simulink model "TestModelWLRover_Script"  (R2023a)
settings: Solver=ode4  StartTime=0.0  StopTime=10  FixedStep=0.0005  RelTol=1e-3
values from neighbouring files (symbols this model uses):
  ADAMS_cwd = 'C:\Users\wfism'    [Controls_Plant_2.m]
  ADAMS_exec = ''    [Controls_Plant_2.m]
  ADAMS_host = 'MSI'    [Controls_Plant_2.m]
  ADAMS_init = ''    [Controls_Plant_2.m]
  ADAMS_inputs = 'hipFLTorque!hipFRTorque!hipMLTorque!hipMRTorque!kneeFLTorque!kneeFRTorque!kneeMLTorque!kneeMRTorque!steerFLTorque!steerFRTorque!steerMLTorque!steerMRTorque!wheelFLTorque!wheelFRTorque!wheelMLTorque!wheelMRTorque'    [Controls_Plant_2.m]
  ADAMS_outputs = 'bodyAcceleration_X!bodyAcceleration_Y!bodyAcceleration_Z!bodyAngle_Pitch!bodyAngle_Roll!bodyAngle_Yaw!bodyAngVelocity_X!bodyAngVelocity_Y!bodyAngVelocity_Z!bodyCoord_X!bodyCoord_Y!bodyCoord_Z!bodyVelocity_X!bodyVelocity_Y!bodyVelocity_Z!hipFLAcceleration!hipFLAngle!hipFLSpeed!hipFRAcceleration!hipFRAngle!hipFRSpeed!hipMLAcceleration!hipMLAngle!hipMLSpeed!hipMRAcceleration!hipMRAngle!hipMRSpeed!kn ...(+718 chars)    [Controls_Plant_2.m]
  ADAMS_prefix = 'Controls_Plant_2'    [Controls_Plant_2.m]
  ADAMS_static = 'no'    [Controls_Plant_2.m]
  ADAMS_sysdir = 'C:\PROGRA~1\MSC~1.SOF\Adams\2019_2\'    [Controls_Plant_2.m]
undefined symbols (not defined in the file or in its folder): roverControllerScript, roverManager, stateWatcher
settings Model: SimulationMode=accelerator  Creator=i.shardyko  LastModifiedBy=a.abramenko
settings OptimizationCC: ReuseModelBlockBuffer=off

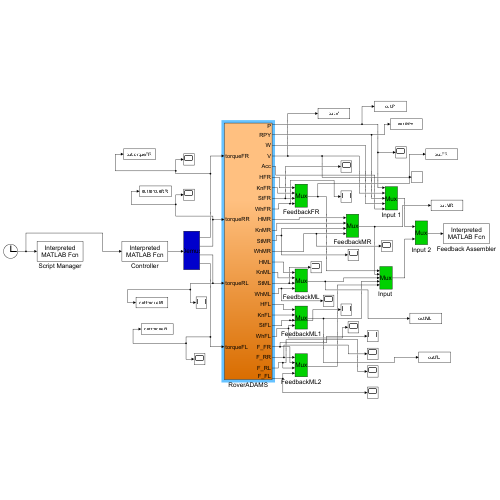
[thumbnail: Simulink's stored preview of the top-level diagram]
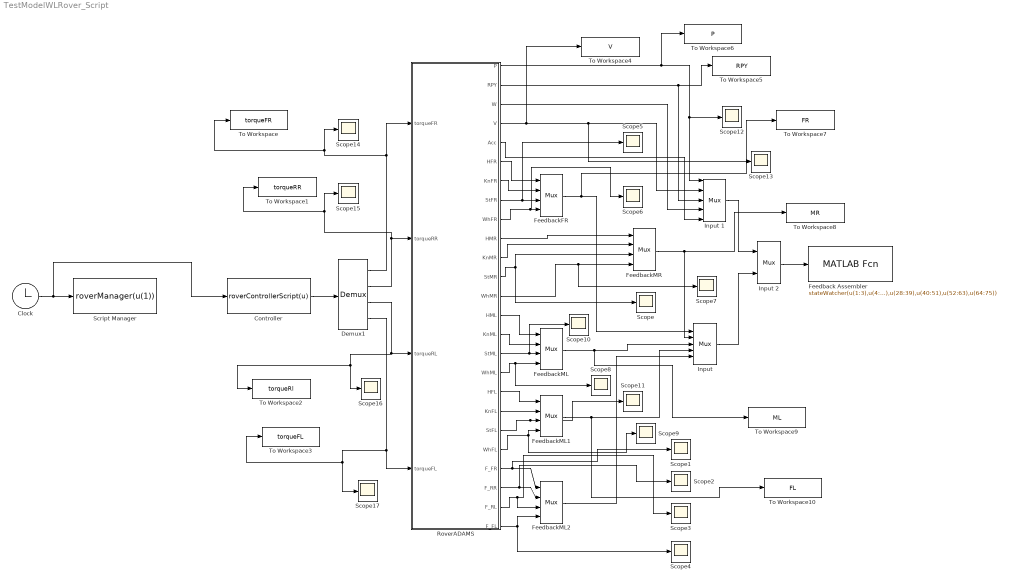
== system TestModelWLRover_Script ==
  Clock : Clock
  Controller : MATLABFcn  MATLABFcn=roverControllerScript(u)  OutputDimensions=16
  Demux1 : Demux
      settings: DisplayOption=none
  Feedback Assembler : MATLABFcn  MATLABFcn=stateWatcher(u(1:3),u(4:6),u(7:9),u(10:12),u(13:15),u(16:27),u(28:39),u(40:51),u(52:63),u(64:75))  OutputDimensions=0
  FeedbackFR : Mux
  FeedbackML : Mux
  FeedbackML1 : Mux
  FeedbackML2 : Mux
  FeedbackMR : Mux
  "Input " : Mux  Inputs=5
  Input 1 : Mux  Inputs=5
  Input 2 : Mux  Inputs=2
  RoverADAMS : Subsystem
  Scope{,1..17} (18 alike) : Scope
  Script Manager : MATLABFcn  MATLABFcn=roverManager(u(1))  OutputDimensions=0
  To Workspace : ToWorkspace  VariableName=torqueFR  SaveFormat=Timeseries  SampleTime=-1
  To Workspace1 : ToWorkspace  VariableName=torqueRR  SaveFormat=Timeseries  SampleTime=-1
  To Workspace10 : ToWorkspace  VariableName=FL  SaveFormat=Timeseries  SampleTime=-1
  To Workspace2 : ToWorkspace  VariableName=torqueRl  SaveFormat=Timeseries  SampleTime=-1
  To Workspace3 : ToWorkspace  VariableName=torqueFL  SaveFormat=Timeseries  SampleTime=-1
  To Workspace4 : ToWorkspace  VariableName=V  SaveFormat=Timeseries  SampleTime=-1
  To Workspace5 : ToWorkspace  VariableName=RPY  SaveFormat=Timeseries  SampleTime=-1
  To Workspace6 : ToWorkspace  VariableName=P  SaveFormat=Timeseries  SampleTime=-1
  To Workspace7 : ToWorkspace  VariableName=FR  SaveFormat=Timeseries  SampleTime=-1
  To Workspace8 : ToWorkspace  VariableName=MR  SaveFormat=Timeseries  SampleTime=-1
  To Workspace9 : ToWorkspace  VariableName=ML  SaveFormat=Timeseries  SampleTime=-1
  wires:
  Controller/1 -> Demux1/1
  Demux1/2 -> To Workspace1/1, Scope15/1, RoverADAMS/2(torqueRR)
  Demux1/3 -> To Workspace2/1, Scope16/1, RoverADAMS/3(torqueRL)
  Demux1/1 -> To Workspace/1, Scope14/1, RoverADAMS/1(torqueFR)
  Demux1/4 -> To Workspace3/1, Scope17/1, RoverADAMS/4(torqueFL)
  RoverADAMS/6(HFR) -> FeedbackFR/1
  RoverADAMS/7(KnFR) -> FeedbackFR/2
  RoverADAMS/8(StFR) -> Scope5/1, FeedbackFR/3
  RoverADAMS/9(WhFR) -> Scope6/1, FeedbackFR/4
  RoverADAMS/10(HMR) -> FeedbackMR/1
  RoverADAMS/11(KnMR) -> FeedbackMR/2
  RoverADAMS/12(StMR) -> FeedbackMR/3, Scope/1
  RoverADAMS/13(WhMR) -> Scope7/1, FeedbackMR/4
  FeedbackMR/1 -> To Workspace8/1, "Input "/2
  RoverADAMS/14(HML) -> FeedbackML/1
  RoverADAMS/15(KnML) -> FeedbackML/2
  RoverADAMS/16(StML) -> Scope10/1, FeedbackML/3
  RoverADAMS/17(WhML) -> FeedbackML/4, Scope8/1
  RoverADAMS/18(HFL) -> FeedbackML1/1
  RoverADAMS/19(KnFL) -> FeedbackML1/2
  RoverADAMS/20(StFL) -> Scope11/1, FeedbackML1/3
  RoverADAMS/21(WhFL) -> FeedbackML1/4, Scope9/1
  FeedbackML/1 -> To Workspace9/1, "Input "/3
  FeedbackML1/1 -> To Workspace10/1, "Input "/4
  RoverADAMS/22(F_FR) -> FeedbackML2/1, Scope1/1
  RoverADAMS/23(F_RR) -> Scope2/1, FeedbackML2/2
  RoverADAMS/24(F_RL) -> Scope3/1, FeedbackML2/3
  RoverADAMS/25(F_FL) -> FeedbackML2/4, Scope4/1
  FeedbackML2/1 -> "Input "/5
  FeedbackFR/1 -> To Workspace7/1, "Input "/1
  Clock/1 -> Controller/1, Script Manager/1
  Input 2/1 -> Feedback Assembler/1
  Input 1/1 -> Input 2/1
  "Input "/1 -> Input 2/2
  RoverADAMS/1(P) -> To Workspace6/1, Scope12/1, Input 1/1
  RoverADAMS/4(V) -> To Workspace4/1, Scope13/1, Input 1/2
  RoverADAMS/2(RPY) -> To Workspace5/1, Input 1/3
  RoverADAMS/3(W) -> Input 1/4
  RoverADAMS/5(Acc) -> Input 1/5

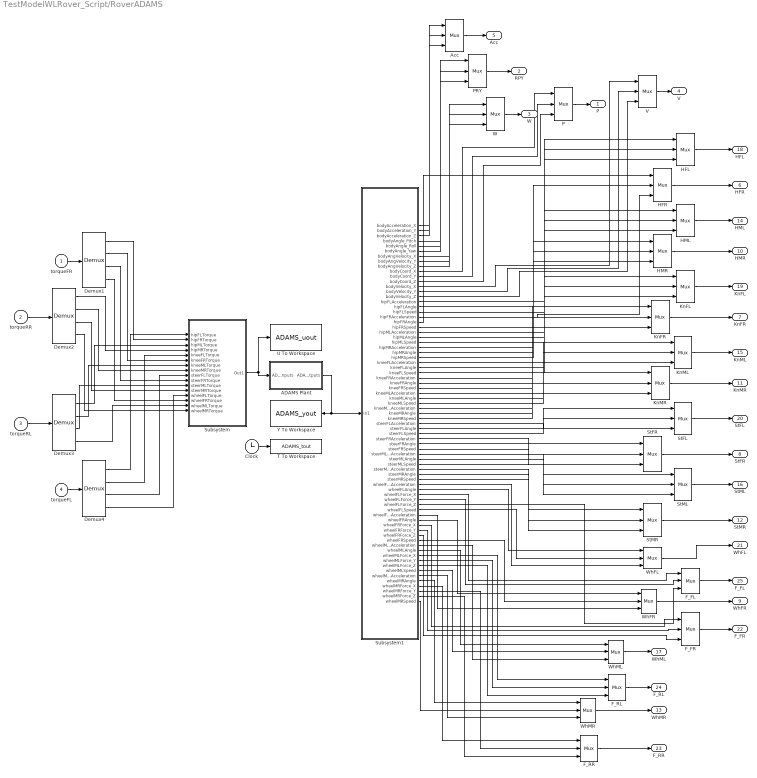
== system TestModelWLRover_Script/RoverADAMS ==
  torqueFR : Inport
  torqueRR : Inport  Port=2
  torqueRL : Inport  Port=3
  torqueFL : Inport  Port=4
  ADAMS Plant : Subsystem  LoadFcn=|  InitFcn=clear mex  mask(Adams Plant){exevie=ADAMS_sysdir, nam_in=ADAMS_inputs, namout=ADAMS_outputs, nampre=ADAMS_prefix, outfil=ADAMS_prefix, exesol=ADAMS_exec, stat=ADAMS_static, inicmd=[ADAMS_init], exetyp=C++, comtyp=PIPE(DDE), workdir=ADAMS_cwd, ada_host=ADAMS_host, modani=interactive, modsim=discrete, dft=no, simulink_lead_cosim=yes, pin_interp_order=0, pout_extrap_order=0, pin_extrap_order=0, pout_interp_order=0, dt_out=0.001, o_rate=1, more=off}
      | %check based on dialog box setting for when setting by popup menu                                             
      | if exist('ADAMS_solver_type')                                                                                 
      |   if strcmp(ADAMS_solver_type,'C++')                                                                          
      |     set_param(gcb,'exetyp','C++');                                                                            
      |   else                                                                                                        
      |     set_param(gcb,'exetyp','Fortran');                                                                        
      |   end                                                                                                         
      | else                                                                                                          
      |   set_param(gcb,'exetyp','C++');                                                                              
      | end                                                                                                           
      | %set the mode if using acar_solver                                                                            
      | %REQUIRED HERE BECAUSE BELOW CAUSES MDLTERMINATE TO BE CALLED 2 TIMES IN MIDDLE OF SIMULATION WHEN SET IN MASK
      |                                                                                                               
      | %enable the direct feedthrough, sim mode, anim mode parameters by default                                     
      |                                                                                                               
      | if exist('set_some_params_states')                                                                            
      |                                                                                                               
      |   set_some_params_states({'dft','modsim','modani'},{'on','on','on'},'MaskEnables',gcb)                        
      |   %turn on direct feedthrough option                                                                          
      |   set_some_params_states({'dft'},{'on'},'MaskVisibilities',gcb)                                               
      |                                                                                                               
      |  end                                                                                                          
      |                                                                                                               
      |                                                                                                               
      | if exist('ADAMS_exec')                                                                                        
      |   if and(strcmp(get_param(gcb,'exesol'),'ADAMS_exec'),strcmp(ADAMS_exec,'acar_solver'))                       
      |     %set the sim mode to discrete -- only supported mode                                                      
      |     set_param(gcb,'modsim','discrete')                                                                        
      |      %turn off direct feedthrough option                                                                      
      |      set_some_params_states({'dft'},{'off'},'MaskVisibilities',gcb)                                           
      |     %set the animation mode to batch -- only supported mode                                                   
      |     set_param(gcb,'modani','batch')                                                                           
      |     %disable the direct feedthrough, sim mode, anim mode parameters                                           
      |     set_some_params_states({'modsim','modani'},{'off','off'},'MaskEnables',gcb)                               
      |   end
      |   if and(strcmp(get_param(gcb,'exesol'),'ADAMS_exec'),strcmp(ADAMS_exec,'apre_solver'))                       
      |     %set the sim mode to discrete -- only supported mode                                                      
      |     set_param(gcb,'modsim','discrete')                                                                        
      |      %turn off direct feedthrough option                                                                      
      |      set_some_params_states({'dft'},{'off'},'MaskVisibilities',gcb)                                           
      |     %set the animation mode to batch -- only supported mode                                                   
      |     set_param(gcb,'modani','batch')                                                                           
      |     %disable the direct feedthrough, sim mode, anim mode parameters                                           
      |     set_some_params_states({'modsim','modani'},{'off','off'},'MaskEnables',gcb)                               
      |   end                                                                                                  
      | end
      mask prompts: exevie "Adams install directory"; nam_in "Adams View input names"; namout "Adams View output names"; nampre "Adams model file prefix"; outfil "Output files prefix (opt.: if blank - no output)"; exesol "User executable (opt.: if blank - use standard)"; stat "Initial static simulation flag"; inicmd "Initialization commands"; exetyp "Adams Solver type"; comtyp "Interprocess option"; workdir "Adams working directory"; ada_host "Adams host"; modani "Animation mode"; modsim "Simulation mode"; dft "Direct feedthrough"; simulink_lead_cosim "Discrete Computational Order - Simulink Leads Adams"; pin_interp_order "Plant input interpolation order"; pout_extrap_order "Plant output extrapolation order"; pin_extrap_order "Plant input extrapolation order"; pout_interp_order "Plant output interpolation order"; dt_out "Communication interval"; o_rate "Number of communications per output step"; more "More parameters"
      mask help: Simulate any Adams plant model either in Adams Solver form (.adm file) or in Adams View form (.cmd file)
      settings: OpenFcn=|
      | open_system(gcb,'mask')
      | if not(exist('set_some_params_states'))
      | 
      | warning('The script "set_some_params_states.m" cannot be found in the MATLAB PATH.  Cannot update the ADAMS Plant S-Function parameters.')
      | 
      | warning('Recommended action(optional):  run the Adams Controls .m file first to help choose the correct settings in the Adams S-Function block.')
      | 
      | end
      mask Help:
      | <html>
      | This S-Function represents the non-linear Adams Plant with the inputs sent to the Adams model <br>
      |  and the outputs generated by the Adams model.  See the Adams Controls documentation for more <br>
      | information.  This plant uses the following variables:<br>
      | <br>
      | <b>ADAMS_sysdir  :</b> Adams installation directory<br>
      | <b>ADAMS_inputs  :</b> Input variables View names vector<br>
      | <b>ADAMS_outputs :</b> Outputs variables View names vector<br>
      | <b>ADAMS_prefix  : </b>ADAMS model files prefix (.adm, .cmd); also doubles as output files prefix<br>
      | <b>ADAMS_exec :</b> Adams Solver user library or keyword (e.g., acar_solver)<br>
      | <b>ADAMS_static :</b> yes|no - initial static before Co-simulation(discrete)/Function Evaluation(continuous)<br>
      | <b>ADAMS_init :</b>Initialization commands (i.e., Adams View or Solver commands, depending on setting for Animation mode)<br>
      | <b>ADAMS_cwd : </b> Current working directory (for TCP/IP)<br>
      | <b>ADAMS_host : </b>Name of Adams server host (for TCP/IP)<br>
      | <b>ADAMS_mode :</b> Linear or non-linear (i.e., co-sim, function eval)<br>
      | <b>ADAMS_solver_type :</b>Fortran or C++ (used to set popup menu when first loaded) <br>
      | 
      | 
      | <br>
      | The following settings can be chosen:<br>
      | <br>
      | <b>Adams Solver type:</b>  Fortran or C++ (will also set ADAMS_solver_type)<br>
      | <b>Interprocess option:</b> Pipe(DDE), TCP/IP or DIRECT; TCP/IP can allow different machines run Adams and MATLAB<br>
      | <b>Animation mode:</b> batch (Solver, uses .adm) or interactive (View, uses .cmd)<br>
      | <b>Simulation mode:</b> discrete (Co-simulation) or continuous (Function Evaluation)<br>
      | <b>Discrete Computational Order - Simulink Lead Adams:</b> for discrete mode, chooses if Simulink leads the integration (yes) or lags (no);<br> if set to "no", can remove algebraic loop<br>
      | <b>Plant input interpolation order:</b> 0 = zero-order hold; 1 = linear (discrete mode only, where Simulink leads)<br>
      | <b>Plant output extrapolation order:</b> 0 = zero-order hold;1 = linear(discrete mode only, where Simulink leads)<br>
      | <b>Plant input extrapolation order:</b> 0 = zero-order hold; 1 = linear (discrete mode only, where Adams leads)<br>
      | <b>Plant output interpolation order:</b> 0 = zero-order hold;1 = linear(discrete mode only, where Adams leads)<br>
      | <b>Direct feedthrough:</b> yes|no - yes = Input directly effect output(continuous mode-only)<br>
      | <b>Communication interval:</b> Time step at which Co-simulation exchange information (e.g.,0.005); also controls <br>output for continuous mode (Function Evaluation)<br>
      | <b>Number of communications per output step: </b>Sets Adams output rate (.res, .req, .gra) integer value (default: 1)<br>
      | </html>
      mask Callback exesol:
      | if exist('set_some_params_states')
      | %enable the direct feedthrough, sim mode, anim mode parameters
      | set_some_params_states({'dft','modsim','modani'},{'on','on','on'},'MaskEnables',gcb)
      | %turn on direct feedthrough option
      | set_some_params_states({'dft'},{'on'},'MaskVisibilities',gcb)
      | end
      | 
      | if exist('ADAMS_exec')
      |   if and(strcmp(get_param(gcb,'exesol'),'ADAMS_exec'),strcmp(ADAMS_exec,'acar_solver'))
      |     %set the sim mode to discrete -- only supported mode
      |     %REMOVED:  BELOW CAUSES MDLTERMINATE TO BE CALLED 2 TIMES IN MIDDLE OF SIMULATION
      |     %Now in LoadFcn callback
      |     %set_param(gcb,'modsim','discrete')
      |      %turn off direct feedthrough option
      |     set_some_params_states({'dft'},{'off'},'MaskVisibilities',gcb)
      |     %set the animation mode to batch -- only supported mode
      |     %REMOVED:  BELOW CAUSES MDLTERMINATE TO BE CALLED 2 TIMES IN MIDDLE OF SIMULATION
      |     %Now in LoadFcn callback
      |     %set_param(gcb,'modani','batch')
      |     %disable the direct feedthrough, sim mode, anim mode parameters
      |     set_some_params_states({'modsim','modani'},{'off','off'},'MaskEnables',gcb)
      |   end
      | end
      mask TypeOptions exetyp: Fortran | C++
      mask Callback exetyp:
      | if strcmp(get_param(gcb,'exetyp'),'C++')
      |     ADAMS_solver_type='C++';
      | else
      |     ADAMS_solver_type='Fortran';
      | end
      mask TypeOptions comtyp: PIPE(DDE) | TCP/IP | DIRECT
      mask Callback comtyp:
      | if exist('set_some_params_states')
      | if strcmp(get_param(gcb,'comtyp'),'PIPE(DDE)') || strcmp(get_param(gcb,'comtyp'),'DIRECT')
      |     %turn off cwd, host options
      |     set_some_params_states({'ada_host','workdir'},{'off','off'},'MaskVisibilities',gcb)
      | else%if strcmp(get_param(gcb,'modsim'),'TCP/IP')
      |     %turn on cwd, host options
      |     set_some_params_states({'ada_host','workdir'},{'on','on'},'MaskVisibilities',gcb)
      | end
      | end
      mask TypeOptions modani: batch | interactive
      mask TypeOptions modsim: discrete | continuous
      mask Callback modsim:
      | if exist('set_some_params_states')
      | if strcmp(get_param(gcb,'modsim'),'discrete')
      |      %turn off direct feedthrough option
      |     set_some_params_states({'dft'},{'off'},'MaskVisibilities',gcb)
      |     %turn on discrete co-sim type if want to see more
      |     if strcmp(get_param(gcb,'more'),'on')
      |         set_some_params_states({'simulink_lead_cosim'},{'on'},'MaskVisibilities',gcb)
      |     end
      |     if strcmp(get_param(gcb,'simulink_lead_cosim'),'yes')
      |         %turn on interpolation/extrapolation options
      |         set_some_params_states({'pin_interp_order','pout_extrap_order',},{'on','on'},'MaskVisibilities',gcb)
      |     else
      |         set_some_params_states({'pin_extrap_order','pout_interp_order'},{'on','on'},'MaskVisibilities',gcb)
      |     end
      | else%if strcmp(get_param(gcb,'modsim'),'continuous')
      |      %turn off direct feedthrough option
      |     set_some_params_states({'dft'},{'on'},'MaskVisibilities',gcb)
      |     %turn off interpolation/extrapolation options
      |     set_some_params_states({'pin_interp_order','pout_extrap_order','pin_extrap_order','pout_interp_order','simulink_lead_cosim'},{'off','off','off','off','off'},'MaskVisibilities',gcb)
      | end
      | end
      mask TypeOptions dft: no | yes
      mask TypeOptions simulink_lead_cosim: yes | no
      mask Callback simulink_lead_cosim:
      | if exist('set_some_params_states')
      | if (strcmp(get_param(gcb,'simulink_lead_cosim'),'yes') && strcmp(get_param(gcb,'modsim'),'discrete'))
      |      %turn off unused interpolate/extrapolate options
      |     set_some_params_states({'pin_extrap_order','pout_interp_order'},{'off','off'},'MaskVisibilities',gcb)
      |     %turn on used interpolate/extrapolate options
      |     set_some_params_states({'pin_interp_order','pout_extrap_order'},{'on','on'},'MaskVisibilities',gcb)
      | elseif (strcmp(get_param(gcb,'simulink_lead_cosim'),'no') && strcmp(get_param(gcb,'modsim'),'discrete'))
      |     %turn on used interpolate/extrapolate options
      |     set_some_params_states({'pin_extrap_order','pout_interp_order'},{'on','on'},'MaskVisibilities',gcb)
      |      %turn off unused interpolate/extrapolate options
      |     set_some_params_states({'pin_interp_order','pout_extrap_order'},{'off','off'},'MaskVisibilities',gcb)
      | end
      | end
      mask TypeOptions pin_interp_order: 0 | 1
      mask TypeOptions pout_extrap_order: 0 | 1
      mask TypeOptions pin_extrap_order: 0 | 1
      mask TypeOptions pout_interp_order: 0 | 1
      mask Callback more:
      | if exist('set_some_params_states')
      | if (strcmp(get_param(gcb,'more'),'on'))
      |      %turn on infrequently used options
      |     set_some_params_states({'exevie','nam_in','namout','exesol','stat','inicmd'},{'on','on','on','on','on','on'},'MaskVisibilities',gcb)
      |     if strcmp(get_param(gcb,'modsim'),'discrete')
      |         set_some_params_states({'simulink_lead_cosim'},{'on'},'MaskVisibilities',gcb)
      |     end
      | elseif (strcmp(get_param(gcb,'more'),'off'))
      |     %turn off infrequently used options
      |     set_some_params_states({'exevie','nam_in','namout','exesol','stat','inicmd'},{'off','off','off','off','off','off'},'MaskVisibilities',gcb)
      |     if strcmp(get_param(gcb,'modsim'),'discrete')
      |         set_some_params_states({'simulink_lead_cosim'},{'off'},'MaskVisibilities',gcb)
      |     end
      | end
      | end
      mask Display: disp( 'MSC Software' )
  "Acc " : Mux  Inputs=3
  Clock : Clock
  Demux{1..4} (4 alike) : Demux
      settings: DisplayOption=none
  "F_FL " : Mux  Inputs=3
  "F_FR " : Mux  Inputs=3
  "F_RL " : Mux  Inputs=3
  "F_RR " : Mux  Inputs=3
  "HFL " : Mux  Inputs=3
  "HFR " : Mux  Inputs=3
  "HML " : Mux  Inputs=3
  "HMR " : Mux  Inputs=3
  "KnFL " : Mux  Inputs=3
  "KnFR " : Mux  Inputs=3
  "KnML " : Mux  Inputs=3
  "KnMR " : Mux  Inputs=3
  "P " : Mux  Inputs=3
  "PRY " : Mux  Inputs=3
  "StFL " : Mux  Inputs=3
  "StFR " : Mux  Inputs=3
  "StML " : Mux  Inputs=3
  "StMR " : Mux  Inputs=3
  Subsystem : Subsystem
  Subsystem1 : Subsystem
  T To Workspace : ToWorkspace  VariableName=ADAMS_tout
      settings: MaxDataPoints=100000
  U To Workspace : ToWorkspace  VariableName=ADAMS_uout
      settings: MaxDataPoints=100000
  "V " : Mux  Inputs=3
  "W " : Mux  Inputs=3
  "WhFL " : Mux  Inputs=3
  "WhFR " : Mux  Inputs=3
  "WhML " : Mux  Inputs=3
  "WhMR " : Mux  Inputs=3
  Y To Workspace : ToWorkspace  VariableName=ADAMS_yout
      settings: MaxDataPoints=100000
  P : Outport
  RPY : Outport  Port=2
  W : Outport  Port=3
  V : Outport  Port=4
  Acc : Outport  Port=5
  HFR : Outport  Port=6
  KnFR : Outport  Port=7
  StFR : Outport  Port=8
  WhFR : Outport  Port=9
  HMR : Outport  Port=10
  KnMR : Outport  Port=11
  StMR : Outport  Port=12
  WhMR : Outport  Port=13
  HML : Outport  Port=14
  KnML : Outport  Port=15
  StML : Outport  Port=16
  WhML : Outport  Port=17
  HFL : Outport  Port=18
  KnFL : Outport  Port=19
  StFL : Outport  Port=20
  WhFL : Outport  Port=21
  F_FR : Outport  Port=22
  F_RR : Outport  Port=23
  F_RL : Outport  Port=24
  F_FL : Outport  Port=25
  wires:
  Subsystem1/40(steerFLAcceleration) -> "StFL "/3
  Demux3/4 -> Subsystem/15(wheelMLTorque)
  Subsystem1/35("kneeMLAngle        ") -> "KnML "/1
  Subsystem1/38("kneeMRAngle        ") -> "KnMR "/1
  "HML "/1 -> HML/1
  Subsystem1/37("kneeMRAcceleration ") -> "KnMR "/3
  Demux2/1 -> Subsystem/4("hipMRTorque  ")
  Demux3/3 -> Subsystem/11(steerMLTorque)
  "StFR "/1 -> StFR/1
  Subsystem1/72("wheelMRForce_X     ") -> "F_RR "/1
  Subsystem1/74("wheelMRForce_Z     ") -> "F_RR "/3
  "StMR "/1 -> StMR/1
  "StFL "/1 -> StFL/1
  Subsystem1/70(wheelMRAcceleration) -> "WhMR "/3
  Subsystem1/65("wheelMLAngle       ") -> "WhML "/1
  Subsystem1/5("bodyAngle_Roll     ") -> "PRY "/2
  "HFL "/1 -> HFL/1
  Subsystem1/39("kneeMRSpeed        ") -> "KnMR "/2
  Subsystem1/51("steerMRSpeed       ") -> "StMR "/2
  Subsystem1/73("wheelMRForce_Y     ") -> "F_RR "/2
  Subsystem1/71("wheelMRAngle       ") -> "WhMR "/1
  torqueFR/1 -> Demux1/1
  "KnMR "/1 -> KnMR/1
  Clock/1 -> T To Workspace/1
  Subsystem1/42("steerFLSpeed       ") -> "StFL "/2
  torqueRL/1 -> Demux3/1
  Subsystem1/41("steerFLAngle       ") -> "StFL "/1
  Demux1/2 -> Subsystem/6("kneeFRTorque ")
  Subsystem1/63("wheelFRSpeed       ") -> "WhFR "/2
  Subsystem1/69("wheelMLSpeed       ") -> "WhML "/2
  Demux4/3 -> Subsystem/9(steerFLTorque)
  Demux1/1 -> Subsystem/2("hipFRTorque  ")
  Subsystem1/13("bodyVelocity_X     ") -> "V "/1
  Subsystem1/36("kneeMLSpeed        ") -> "KnML "/2
  Subsystem1/75("wheelMRSpeed       ") -> "WhMR "/2
  "WhML "/1 -> WhML/1
  Subsystem1/44("steerFRAngle       ") -> "StFR "/1
  Demux3/1 -> Subsystem/3("hipMLTorque  ")
  Subsystem1/56("wheelFLForce_Z     ") -> "F_FL "/3
  Demux4/1 -> Subsystem/1("hipFLTorque  ")
  Subsystem1/33("kneeFRSpeed        ") -> "KnFR "/2
  Subsystem1/27("hipMRSpeed         ") -> "HMR "/2
  Demux2/2 -> Subsystem/8("kneeMRTorque ")
  Demux3/2 -> Subsystem/7("kneeMLTorque ")
  "HFR "/1 -> HFR/1
  Subsystem/1(Out1) -> ADAMS Plant/1(ADAMS inputs), U To Workspace/1
  Subsystem1/59("wheelFRAngle       ") -> "WhFR "/1
  Demux1/3 -> Subsystem/10(steerFRTorque)
  Subsystem1/57("wheelFLSpeed       ") -> "WhFL "/2
  ADAMS Plant/1(ADAMS outputs) -> Subsystem1/1(In1), Y To Workspace/1
  Subsystem1/29("kneeFLAngle        ") -> "KnFL "/1
  Demux1/4 -> Subsystem/14(wheelFRTorque)
  Subsystem1/61("wheelFRForce_Y     ") -> "F_FR "/2
  "PRY "/1 -> RPY/1
  Demux2/4 -> Subsystem/16(wheelMRTorque)
  "KnML "/1 -> KnML/1
  Demux4/4 -> Subsystem/13(wheelFLTorque)
  Subsystem1/49(steerMRAcceleration) -> "StMR "/3
  "KnFR "/1 -> KnFR/1
  Subsystem1/62("wheelFRForce_Z     ") -> "F_FR "/3
  "WhFL "/1 -> WhFL/1
  Demux2/3 -> Subsystem/12(steerMRTorque)
  "P "/1 -> P/1
  Subsystem1/50("steerMRAngle       ") -> "StMR "/1
  "KnFL "/1 -> KnFL/1
  Subsystem1/32("kneeFRAngle        ") -> "KnFR "/1
  Subsystem1/28("kneeFLAcceleration ") -> "KnFL "/3
  Subsystem1/66("wheelMLForce_X     ") -> "F_RL "/1
  "V "/1 -> V/1
  Subsystem1/46(steerMLAcceleration) -> "StML "/3
  Subsystem1/58(wheelFRAcceleration) -> "WhFR "/3
  torqueRR/1 -> Demux2/1
  Subsystem1/67("wheelMLForce_Y     ") -> "F_RL "/2
  Subsystem1/64(wheelMLAcceleration) -> "WhML "/3
  Subsystem1/9("bodyAngVelocity_Z  ") -> "W "/3
  Subsystem1/14("bodyVelocity_Y     ") -> "V "/2
  Subsystem1/31("kneeFRAcceleration ") -> "KnFR "/3
  Subsystem1/8("bodyAngVelocity_Y  ") -> "W "/2
  Subsystem1/11("bodyCoord_Y        ") -> "P "/2
  Subsystem1/68("wheelMLForce_Z     ") -> "F_RL "/3
  Subsystem1/10("bodyCoord_X        ") -> "P "/1
  Subsystem1/12("bodyCoord_Z        ") -> "P "/3
  Subsystem1/4("bodyAngle_Pitch    ") -> "PRY "/1
  Subsystem1/24("hipMLSpeed         ") -> "HML "/2
  Subsystem1/26("hipMRAngle         ") -> "HMR "/1
  Subsystem1/55("wheelFLForce_Y     ") -> "F_FL "/2
  Subsystem1/60("wheelFRForce_X     ") -> "F_FR "/1
  Subsystem1/22("hipMLAcceleration  ") -> "HML "/3
  Subsystem1/34("kneeMLAcceleration ") -> "KnML "/3
  Subsystem1/23("hipMLAngle         ") -> "HML "/1
  Subsystem1/25("hipMRAcceleration  ") -> "HMR "/3
  Subsystem1/21("hipFRSpeed         ") -> "HFR "/2
  Subsystem1/20("hipFRAngle         ") -> "HFR "/1
  Subsystem1/53("wheelFLAngle       ") -> "WhFL "/1
  Subsystem1/47("steerMLAngle       ") -> "StML "/1
  Subsystem1/30("kneeFLSpeed        ") -> "KnFL "/2
  Subsystem1/17("hipFLAngle         ") -> "HFL "/1
  Subsystem1/19("hipFRAcceleration  ") -> "HFR "/3
  Subsystem1/18("hipFLSpeed         ") -> "HFL "/2
  Subsystem1/16("hipFLAcceleration  ") -> "HFL "/3
  Subsystem1/1("bodyAcceleration_X ") -> "Acc "/1
  Subsystem1/6("bodyAngle_Yaw      ") -> "PRY "/3
  Subsystem1/15("bodyVelocity_Z     ") -> "V "/3
  Subsystem1/7("bodyAngVelocity_X  ") -> "W "/1
  Subsystem1/3("bodyAcceleration_Z ") -> "Acc "/3
  Subsystem1/2("bodyAcceleration_Y ") -> "Acc "/2
  "Acc "/1 -> Acc/1
  Subsystem1/54("wheelFLForce_X     ") -> "F_FL "/1
  "WhFR "/1 -> WhFR/1
  Subsystem1/48("steerMLSpeed       ") -> "StML "/2
  torqueFL/1 -> Demux4/1
  "WhMR "/1 -> WhMR/1
  Subsystem1/52(wheelFLAcceleration) -> "WhFL "/3
  Subsystem1/43(steerFRAcceleration) -> "StFR "/3
  Subsystem1/45("steerFRSpeed       ") -> "StFR "/2
  Demux4/2 -> Subsystem/5("kneeFLTorque ")
  "StML "/1 -> StML/1
  "W "/1 -> W/1
  "HMR "/1 -> HMR/1
  "F_FR "/1 -> F_FR/1
  "F_RR "/1 -> F_RR/1
  "F_RL "/1 -> F_RL/1
  "F_FL "/1 -> F_FL/1

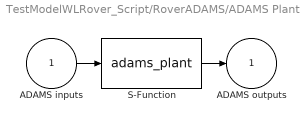
== system TestModelWLRover_Script/RoverADAMS/ADAMS Plant ==
  ADAMS inputs : Inport
  S-Function : S-Function  StopFcn=clear mex  FunctionName=adams_plant  Parameters=exevie,exesol,stat,outfil,nampre,o_rate,nam_in,namout,dft,modsim,modani,dt_out,inicmd,exetyp,comtyp,ada_host, workdir,pin_interp_order,pout_extrap_order,pin_extrap_order,pout_interp_order,simulink_lead_cosim  SFunctionDeploymentMode=off  EnableBusSupport=off
  ADAMS outputs : Outport  InitialOutput=0
  wires:
  ADAMS inputs/1 -> S-Function/1
  S-Function/1 -> ADAMS outputs/1

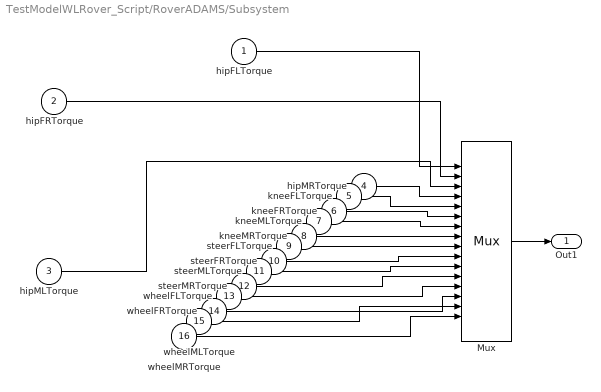
== system TestModelWLRover_Script/RoverADAMS/Subsystem ==
  "hipFLTorque  " : Inport
  "hipFRTorque  " : Inport  Port=2
  "hipMLTorque  " : Inport  Port=3
  "hipMRTorque  " : Inport  Port=4
  "kneeFLTorque " : Inport  Port=5
  "kneeFRTorque " : Inport  Port=6
  "kneeMLTorque " : Inport  Port=7
  "kneeMRTorque " : Inport  Port=8
  steerFLTorque : Inport  Port=9
  steerFRTorque : Inport  Port=10
  steerMLTorque : Inport  Port=11
  steerMRTorque : Inport  Port=12
  wheelFLTorque : Inport  Port=13
  wheelFRTorque : Inport  Port=14
  wheelMLTorque : Inport  Port=15
  wheelMRTorque : Inport  Port=16
  Mux : Mux  Inputs=16
  Out1 : Outport
  wires:
  "hipFLTorque  "/1 -> Mux/1
  "hipMRTorque  "/1 -> Mux/4
  "hipFRTorque  "/1 -> Mux/2
  steerMLTorque/1 -> Mux/11
  "kneeFLTorque "/1 -> Mux/5
  "kneeMRTorque "/1 -> Mux/8
  "kneeMLTorque "/1 -> Mux/7
  "kneeFRTorque "/1 -> Mux/6
  steerFLTorque/1 -> Mux/9
  wheelFLTorque/1 -> Mux/13
  steerFRTorque/1 -> Mux/10
  steerMRTorque/1 -> Mux/12
  wheelMLTorque/1 -> Mux/15
  "hipMLTorque  "/1 -> Mux/3
  wheelMRTorque/1 -> Mux/16
  wheelFRTorque/1 -> Mux/14
  Mux/1 -> Out1/1

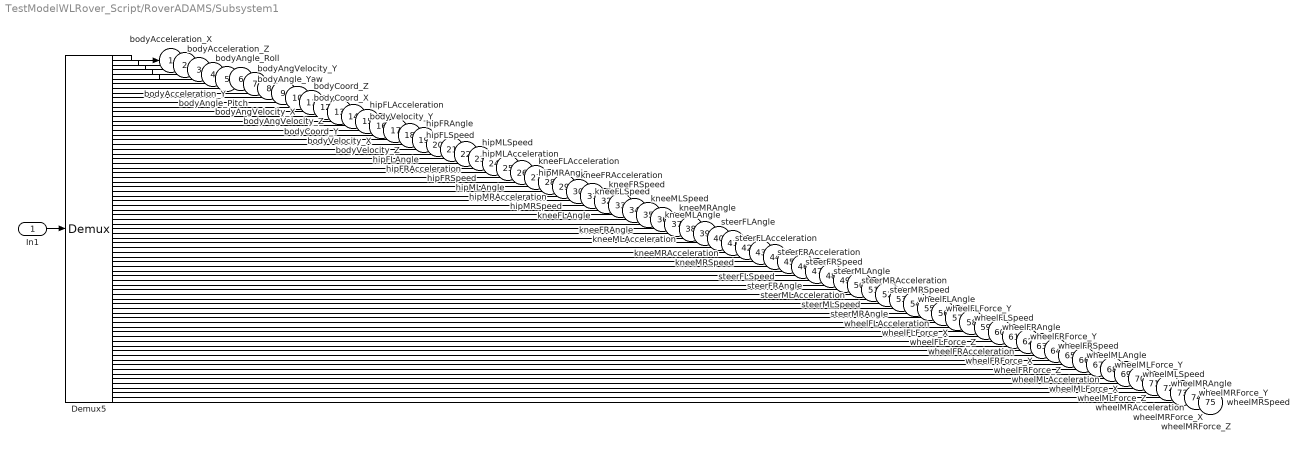
== system TestModelWLRover_Script/RoverADAMS/Subsystem1 ==
  In1 : Inport
  Demux5 : Demux  Outputs=75
      settings: DisplayOption=none
  "bodyAcceleration_X " : Outport
  "bodyAcceleration_Y " : Outport  Port=2
  "bodyAcceleration_Z " : Outport  Port=3
  "bodyAngle_Pitch    " : Outport  Port=4
  "bodyAngle_Roll     " : Outport  Port=5
  "bodyAngle_Yaw      " : Outport  Port=6
  "bodyAngVelocity_X  " : Outport  Port=7
  "bodyAngVelocity_Y  " : Outport  Port=8
  "bodyAngVelocity_Z  " : Outport  Port=9
  "bodyCoord_X        " : Outport  Port=10
  "bodyCoord_Y        " : Outport  Port=11
  "bodyCoord_Z        " : Outport  Port=12
  "bodyVelocity_X     " : Outport  Port=13
  "bodyVelocity_Y     " : Outport  Port=14
  "bodyVelocity_Z     " : Outport  Port=15
  "hipFLAcceleration  " : Outport  Port=16
  "hipFLAngle         " : Outport  Port=17
  "hipFLSpeed         " : Outport  Port=18
  "hipFRAcceleration  " : Outport  Port=19
  "hipFRAngle         " : Outport  Port=20
  "hipFRSpeed         " : Outport  Port=21
  "hipMLAcceleration  " : Outport  Port=22
  "hipMLAngle         " : Outport  Port=23
  "hipMLSpeed         " : Outport  Port=24
  "hipMRAcceleration  " : Outport  Port=25
  "hipMRAngle         " : Outport  Port=26
  "hipMRSpeed         " : Outport  Port=27
  "kneeFLAcceleration " : Outport  Port=28
  "kneeFLAngle        " : Outport  Port=29
  "kneeFLSpeed        " : Outport  Port=30
  "kneeFRAcceleration " : Outport  Port=31
  "kneeFRAngle        " : Outport  Port=32
  "kneeFRSpeed        " : Outport  Port=33
  "kneeMLAcceleration " : Outport  Port=34
  "kneeMLAngle        " : Outport  Port=35
  "kneeMLSpeed        " : Outport  Port=36
  "kneeMRAcceleration " : Outport  Port=37
  "kneeMRAngle        " : Outport  Port=38
  "kneeMRSpeed        " : Outport  Port=39
  steerFLAcceleration : Outport  Port=40
  "steerFLAngle       " : Outport  Port=41
  "steerFLSpeed       " : Outport  Port=42
  steerFRAcceleration : Outport  Port=43
  "steerFRAngle       " : Outport  Port=44
  "steerFRSpeed       " : Outport  Port=45
  steerMLAcceleration : Outport  Port=46
  "steerMLAngle       " : Outport  Port=47
  "steerMLSpeed       " : Outport  Port=48
  steerMRAcceleration : Outport  Port=49
  "steerMRAngle       " : Outport  Port=50
  "steerMRSpeed       " : Outport  Port=51
  wheelFLAcceleration : Outport  Port=52
  "wheelFLAngle       " : Outport  Port=53
  "wheelFLForce_X     " : Outport  Port=54
  "wheelFLForce_Y     " : Outport  Port=55
  "wheelFLForce_Z     " : Outport  Port=56
  "wheelFLSpeed       " : Outport  Port=57
  wheelFRAcceleration : Outport  Port=58
  "wheelFRAngle       " : Outport  Port=59
  "wheelFRForce_X     " : Outport  Port=60
  "wheelFRForce_Y     " : Outport  Port=61
  "wheelFRForce_Z     " : Outport  Port=62
  "wheelFRSpeed       " : Outport  Port=63
  wheelMLAcceleration : Outport  Port=64
  "wheelMLAngle       " : Outport  Port=65
  "wheelMLForce_X     " : Outport  Port=66
  "wheelMLForce_Y     " : Outport  Port=67
  "wheelMLForce_Z     " : Outport  Port=68
  "wheelMLSpeed       " : Outport  Port=69
  wheelMRAcceleration : Outport  Port=70
  "wheelMRAngle       " : Outport  Port=71
  "wheelMRForce_X     " : Outport  Port=72
  "wheelMRForce_Y     " : Outport  Port=73
  "wheelMRForce_Z     " : Outport  Port=74
  "wheelMRSpeed       " : Outport  Port=75
  wires:
  Demux5/72 -> "wheelMRForce_X     "/1
  Demux5/55 -> "wheelFLForce_Y     "/1
  Demux5/63 -> "wheelFRSpeed       "/1
  Demux5/49 -> steerMRAcceleration/1
  Demux5/17 -> "hipFLAngle         "/1
  Demux5/48 -> "steerMLSpeed       "/1
  Demux5/30 -> "kneeFLSpeed        "/1
  Demux5/39 -> "kneeMRSpeed        "/1
  Demux5/42 -> "steerFLSpeed       "/1
  Demux5/64 -> wheelMLAcceleration/1
  Demux5/53 -> "wheelFLAngle       "/1
  Demux5/40 -> steerFLAcceleration/1
  Demux5/59 -> "wheelFRAngle       "/1
  Demux5/44 -> "steerFRAngle       "/1
  Demux5/23 -> "hipMLAngle         "/1
  Demux5/2 -> "bodyAcceleration_Y "/1
  Demux5/54 -> "wheelFLForce_X     "/1
  Demux5/1 -> "bodyAcceleration_X "/1
  Demux5/43 -> steerFRAcceleration/1
  Demux5/36 -> "kneeMLSpeed        "/1
  Demux5/34 -> "kneeMLAcceleration "/1
  Demux5/15 -> "bodyVelocity_Z     "/1
  Demux5/3 -> "bodyAcceleration_Z "/1
  Demux5/74 -> "wheelMRForce_Z     "/1
  Demux5/41 -> "steerFLAngle       "/1
  Demux5/50 -> "steerMRAngle       "/1
  Demux5/70 -> wheelMRAcceleration/1
  Demux5/16 -> "hipFLAcceleration  "/1
  Demux5/52 -> wheelFLAcceleration/1
  Demux5/14 -> "bodyVelocity_Y     "/1
  Demux5/8 -> "bodyAngVelocity_Y  "/1
  Demux5/56 -> "wheelFLForce_Z     "/1
  Demux5/9 -> "bodyAngVelocity_Z  "/1
  Demux5/45 -> "steerFRSpeed       "/1
  Demux5/31 -> "kneeFRAcceleration "/1
  Demux5/29 -> "kneeFLAngle        "/1
  Demux5/21 -> "hipFRSpeed         "/1
  Demux5/35 -> "kneeMLAngle        "/1
  Demux5/68 -> "wheelMLForce_Z     "/1
  Demux5/19 -> "hipFRAcceleration  "/1
  Demux5/12 -> "bodyCoord_Z        "/1
  Demux5/28 -> "kneeFLAcceleration "/1
  Demux5/5 -> "bodyAngle_Roll     "/1
  Demux5/32 -> "kneeFRAngle        "/1
  Demux5/62 -> "wheelFRForce_Z     "/1
  Demux5/58 -> wheelFRAcceleration/1
  Demux5/57 -> "wheelFLSpeed       "/1
  Demux5/38 -> "kneeMRAngle        "/1
  Demux5/4 -> "bodyAngle_Pitch    "/1
  Demux5/46 -> steerMLAcceleration/1
  Demux5/60 -> "wheelFRForce_X     "/1
  Demux5/47 -> "steerMLAngle       "/1
  Demux5/75 -> "wheelMRSpeed       "/1
  Demux5/7 -> "bodyAngVelocity_X  "/1
  Demux5/33 -> "kneeFRSpeed        "/1
  Demux5/27 -> "hipMRSpeed         "/1
  Demux5/11 -> "bodyCoord_Y        "/1
  Demux5/66 -> "wheelMLForce_X     "/1
  Demux5/65 -> "wheelMLAngle       "/1
  Demux5/26 -> "hipMRAngle         "/1
  Demux5/6 -> "bodyAngle_Yaw      "/1
  Demux5/69 -> "wheelMLSpeed       "/1
  Demux5/18 -> "hipFLSpeed         "/1
  Demux5/71 -> "wheelMRAngle       "/1
  Demux5/61 -> "wheelFRForce_Y     "/1
  Demux5/20 -> "hipFRAngle         "/1
  Demux5/73 -> "wheelMRForce_Y     "/1
  Demux5/37 -> "kneeMRAcceleration "/1
  Demux5/25 -> "hipMRAcceleration  "/1
  Demux5/51 -> "steerMRSpeed       "/1
  Demux5/22 -> "hipMLAcceleration  "/1
  Demux5/10 -> "bodyCoord_X        "/1
  Demux5/13 -> "bodyVelocity_X     "/1
  Demux5/24 -> "hipMLSpeed         "/1
  Demux5/67 -> "wheelMLForce_Y     "/1
  In1/1 -> Demux5/1
